simulink model "PVAndBatteryIntegratedPlantForBlackStart_SPS"  (R2024b)
settings: Solver=FixedStepAuto  StartTime=0.0  StopTime=tsim  FixedStep=Ts  RelTol=1e-9  AbsTol=1e-7
InitFcn:
  | %% Black Start Sequence
  | t0 = 0; % Battery IBR initial time
  | t1 = 0.5; % PV IBR initial time
  | t2 = 0.8; % Two IBR sync time
  | t3 = 1.2; % Additional motor load connect
  | t4 = 1.5; % Grid reconnection
  | tsim = 3.0; % Total simulation time
  | 
  | %% System Parameters
  | Vdc = 400;
  | Vnom = 100;
  | Prated = 10000;
  | Qrated = 0;
  | Srated = sqrt(Prated^2+Qrated^2);
  | wnom = 2*pi*60;
  | fnom = 60;
  | 
  | %% VOC Parameters
  | kv = Vnom;
  | ki = 3*Vnom/Srated;
  | Vminpu = 0.95;
  | dwmax = 0.5*2*pi;
  | trisemax = 0.1;
  | 
  | C = 1/sqrt(2)/Vminpu^2/dwmax;
  | L = 1/C/wnom^2;
  | tau = C/kv/ki;
  | epsilon = sqrt(L/C);
  | ksy = 3/2/trisemax;
  | 
  | V_voc_1 = 0;
  | V_voc_2 = 0;
  | 
  | %% Filter Parameters
  | Rf = 0.05;
  | Lf = 500e-6;
  | fsw = 10e3;
  | Ts = 1e-6;
  | 
  | %% Load Parameters
  | Rl = 3*Vnom^2/Prated;
  | Rl1 = Rl;
  | Rl2 = 2*Rl;
  | Rl3 = 20*Rl;
  | 
  | %% DCDC Converter Parameters
  | Kp_V = 1;
  | Ki_V = 10;
  | Imax = 110;
  | Kp_I = 0.0001;
  | Ki_I = 1;
  | Vcmax = 1;
undefined symbols (not defined in the file): C_voc, L_voc, Ll, R_voc
libraries: spsThreePhaseVIMeasurementLib x8, eeTransforms x7, spsHalfBridgeConverterLib x6, spsThreePhaseBreakerLib x6, spsThreePhaseSeriesRLCBranchLib x5, spsControlledCurrentSourceLib x4, spsControlledVoltageSourceLib x4, spsParallelRLCBranchLib x4, spsCurrentMeasurementLib x3, spsVoltageMeasurementLib x3, spsGroundLib x3, spsPower3phInstantaneousLib x3
(part 1 of 2)
settings Model: SimulationMode=accelerator  Creator=marco  LastModifiedBy=wang.shum
settings DebuggingCC: AlgebraicLoopMsg=none
settings RTWCC: GPUComputeCapability=3.5

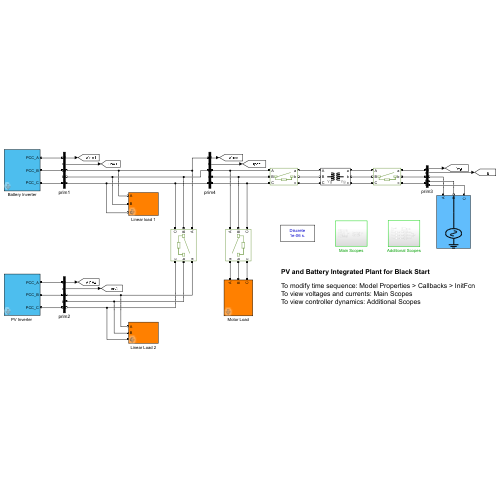
[thumbnail: Simulink's stored preview of the top-level diagram]
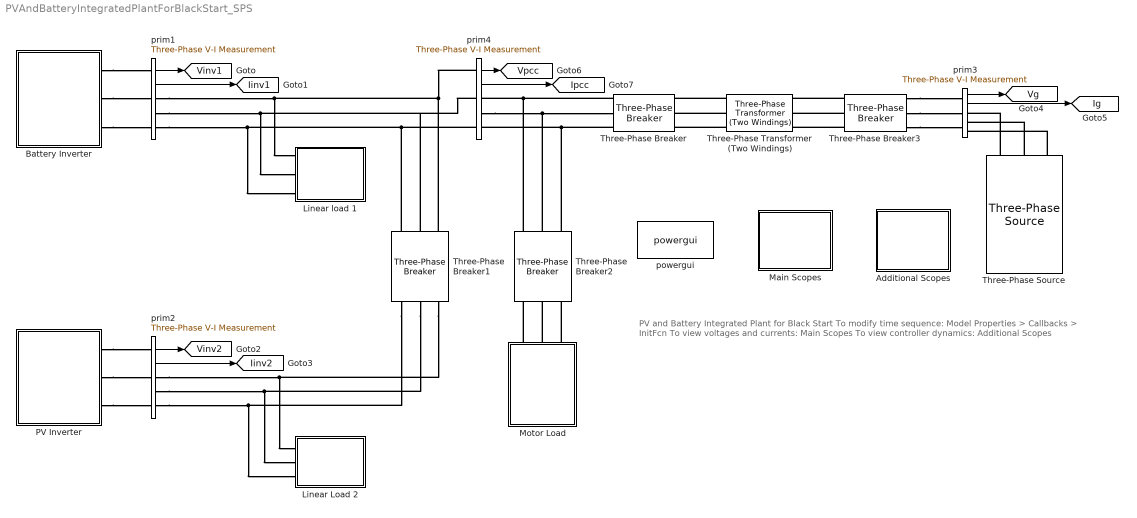
== system PVAndBatteryIntegratedPlantForBlackStart_SPS ==
  note: PV and Battery Integrated Plant for Black Start
      |
      | To modify time sequence: Model Properties > Callbacks > InitFcn
      | To view voltages and currents: Main Scopes
      | To view controller dynamics: Additional Scopes
  Additional Scopes : Subsystem
  Battery Inverter : Subsystem  mask{Vdc=Vdc, Prated=Prated, Qrated=Qrated, t0=t0}
      mask prompts: Vdc "DC Voltage"; Prated "Rated Active Power"; Qrated "Rated Reactive Power"; t0 "Enable Time"
      mask DialogControl DescTextVar Prompt: This block implements an inverter-based resource based on ideal DC source.
      mask DialogControl ParameterGroupVar Prompt: Converter Parameters
      mask DialogControl Container3 Prompt: Controller Parameters
  Linear Load 2 : Subsystem  mask{Rl2=Rl2}
      mask prompts: Rl2 "Load Resistance"
      mask DialogControl DescTextVar Prompt: This is a linear load.
  Linear load 1 : Subsystem  mask{Rl1=Rl1}
      mask prompts: Rl1 "Load Resistance"
      mask DialogControl DescTextVar Prompt: This is a linear load.
  Main Scopes : Subsystem
  Motor Load : Subsystem  mask{Rl3=Rl3, Pm=0}
      mask prompts: Rl3 "Load Resistance"; Pm "Motor Mechanical Power"
      mask DialogControl DescTextVar Prompt: This is an additional load, composed of a linear load and a motor load.
  "PV Inverter " : Subsystem  mask{Vdc=Vdc, Prated=Prated, Qrated=Qrated, t1=t1}
      mask prompts: Vdc "DC Bus Voltage"; Prated "Rated Active Power"; Qrated "Rated Reactive Power"; t1 "Enable Time"
      mask DialogControl DescTextVar Prompt: This block implements an inverter-based resource based on PV source.
      mask DialogControl ParameterGroupVar Prompt: Converter Parameters
      mask DialogControl Container3 Prompt: Controller Parameters
  Three-Phase Transformer (Two Windings) : spsThreePhaseTransformerTwoWindingsLib/Three-Phase Transformer (Two Windings)  Winding1Connection=Yg  Winding2Connection=Yg  CoreType=Three single-phase transformers  SetSaturation=off  Hysteresis=off  DataFile='hysteresis'  SetInitialFlux=off  Measurements=None  UNITS=pu  NominalPower=[ 25e3 , 60 ]  Winding1=[ 122.5 , 0.002 , 0.08 ]  Winding2=[ 122.5 , 0.002 , 0.08 ]  Rm=500  Lm=500  L0=0.5  Saturation=[ 0,0 ; 0.0024,1.2 ; 1.0,1.52 ]  InitialFluxes=[ 0.8 , -0.8 , 0.7 ]  BreakLoop=off  DiscreteSolver=Trapezoidal iterative  DataType=off  TransfoNumber=1
  Three-Phase Breaker : spsThreePhaseBreakerLib/Three-Phase Breaker  InitialState=open  SwitchA=on  SwitchB=on  SwitchC=on  SwitchTimes=t4  External=off  BreakerResistance=0.001  SnubberResistance=1e6  SnubberCapacitance=inf  Measurements=None
  Three-Phase Breaker1 : spsThreePhaseBreakerLib/Three-Phase Breaker  InitialState=open  SwitchA=on  SwitchB=on  SwitchC=on  SwitchTimes=t2  External=off  BreakerResistance=0.001  SnubberResistance=1e6  SnubberCapacitance=inf  Measurements=None
  Three-Phase Breaker2 : spsThreePhaseBreakerLib/Three-Phase Breaker  InitialState=open  SwitchA=on  SwitchB=on  SwitchC=on  SwitchTimes=t3  External=off  BreakerResistance=0.001  SnubberResistance=1e9  SnubberCapacitance=inf  Measurements=None
  Three-Phase Breaker3 : spsThreePhaseBreakerLib/Three-Phase Breaker  InitialState=open  SwitchA=on  SwitchB=on  SwitchC=on  SwitchTimes=t4  External=off  BreakerResistance=0.001  SnubberResistance=1e6  SnubberCapacitance=inf  Measurements=None
  Three-Phase Source : spsThreePhaseSourceLib/Three-Phase Source  InternalConnection=Yg  VoltagePhases=off  Voltage=Vnom*sqrt(3)  PhaseAngle=0  Voltage_phases=[25e3 25e3 25e3]/sqrt(3)  PhaseAngles_phases=[0 -120 +120]  Frequency=fnom  NonIdealSource=on  SpecifyImpedance=off  Resistance=0  Inductance=0  ShortCircuitLevel=100e6  BaseVoltage=Vnom*sqrt(3)  XRratio=7  BusType=swing  Pref=10e3  Qref=0  Prefabc=[10e3, 10e3, 10e3]  Qrefabc=[0, 0, 0]  Qmin=-inf  Qmax=inf
  powergui : sps_lib/powergui  Priority=1  SimulationMode=Discrete  SampleTime=Ts  frequency=60  Iterations=50  frequencyindice=0  Pbase=100e6  ErrMax=1e-4  UnitsV=kV  UnitsW=MW  buscounter=0  FunctionMessages=off  echomessages=off  EnableUseOfTLC=off  CurrentSourceSwitches=off  DisableSnubberDevices=off  DisableRonSwitches=off  DisableVfSwitches=off  DisplayEquations=off  AutomaticDiscreteSolvers=off  SolverType=Tustin/Backward Euler (TBE)  Interpol=off  ExternalGateDelay=off  methode=off  Ts=100  x0status=blocks  SPID=on  SwTol=0  HookPort=off  NonlinearTolerance=1e-4  nMaxIteration=100  ContinueOnMaxIteration=off  RestoreLinks=warning  ResistiveCurrentMeasurement=off  Frange=[0:2:500]  Ylog=off  Xlog=on  ShowGrid=off  save=off  variable=ZData  structure=0  ZoomFFT=off  StartTime=0.0  cycles=1  DisplayStyle=1  fundamental=60  FreqAxis=off  MaxFrequency=1000  frequencyindicesteady=1  RmsSteady=1  display=off
  prim{1..4} (4 alike) : spsThreePhaseVIMeasurementLib/Three-Phase V-I Measurement  VoltageMeasurement=phase-to-ground  SetLabelV=off  LabelV=Vabc_B1  Vpu=off  VpuLL=off  CurrentMeasurement=yes  SetLabelI=off  LabelI=Iabc_B1  Ipu=off  Pbase=100e6  Vbase=500e3  OutputType=Magnitude  PhasorSimulation=off  PSBequivalent=0
  tag scope: Ig=global, Iinv1=global, Iinv2=global, Ipcc=global, Vg=global, Vinv1=global, Vinv2=global, Vpcc=global
  wires:
  prim1/1 -> [Vinv1]
  prim1/2 -> [Iinv1]
  prim3/1 -> [Vg]
  prim3/2 -> [Ig]
  prim2/2 -> [Iinv2]
  prim2/1 -> [Vinv2]
  prim4/1 -> [Vpcc]
  prim4/2 -> [Ipcc]
  connections:
  Battery Inverter/RConn1 -- prim1/LConn1
  Battery Inverter/RConn2 -- prim1/LConn2
  Battery Inverter/RConn3 -- prim1/LConn3
  Three-Phase Breaker1/LConn3 -- prim4/LConn3 -- prim1/RConn3 -- Linear load 1/LConn3
  prim2/RConn1 -- Three-Phase Breaker1/RConn1 -- Linear Load 2/LConn1
  prim2/RConn3 -- Three-Phase Breaker1/RConn3 -- Linear Load 2/LConn3
  "PV Inverter "/RConn3 -- prim2/LConn3
  "PV Inverter "/RConn2 -- prim2/LConn2
  "PV Inverter "/RConn1 -- prim2/LConn1
  Three-Phase Source/RConn1 -- prim3/RConn1
  Three-Phase Source/RConn2 -- prim3/RConn2
  Three-Phase Source/RConn3 -- prim3/RConn3
  Three-Phase Transformer (Two Windings)/LConn2 -- Three-Phase Breaker/RConn2
  Three-Phase Transformer (Two Windings)/LConn1 -- Three-Phase Breaker/RConn1
  Three-Phase Transformer (Two Windings)/LConn3 -- Three-Phase Breaker/RConn3
  Three-Phase Breaker3/RConn2 -- prim3/LConn2
  Three-Phase Breaker3/RConn1 -- prim3/LConn1
  Three-Phase Breaker3/LConn1 -- Three-Phase Transformer (Two Windings)/RConn1
  Three-Phase Breaker3/LConn2 -- Three-Phase Transformer (Two Windings)/RConn2
  Three-Phase Breaker3/LConn3 -- Three-Phase Transformer (Two Windings)/RConn3
  Motor Load/LConn1 -- Three-Phase Breaker2/RConn1
  Motor Load/LConn2 -- Three-Phase Breaker2/RConn2
  Motor Load/LConn3 -- Three-Phase Breaker2/RConn3
  Three-Phase Breaker1/LConn1 -- prim4/LConn1 -- prim1/RConn1 -- Linear load 1/LConn1
  prim2/RConn2 -- Three-Phase Breaker1/RConn2 -- Linear Load 2/LConn2
  Three-Phase Breaker3/RConn3 -- prim3/LConn3
  prim1/RConn2 -- prim4/LConn2 -- Three-Phase Breaker1/LConn2 -- Linear load 1/LConn2
  Three-Phase Breaker2/LConn1 -- Three-Phase Breaker/LConn1 -- prim4/RConn1
  prim4/RConn2 -- Three-Phase Breaker/LConn2 -- Three-Phase Breaker2/LConn2
  Three-Phase Breaker/LConn3 -- prim4/RConn3 -- Three-Phase Breaker2/LConn3

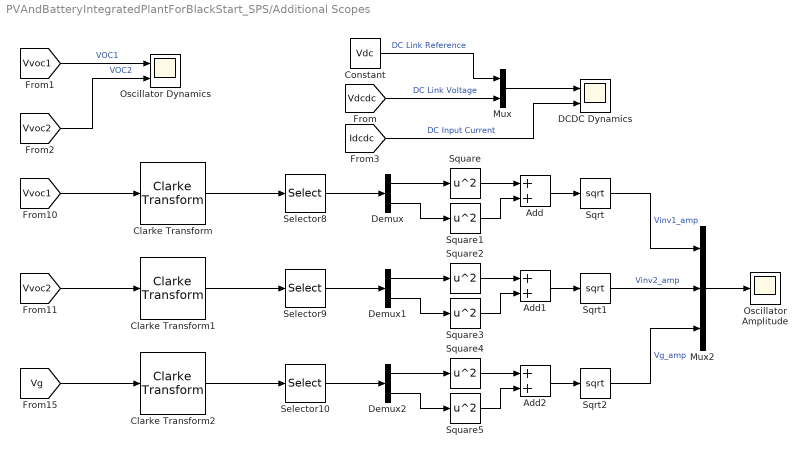
== system PVAndBatteryIntegratedPlantForBlackStart_SPS/Additional Scopes ==
  Add : Sum
  Add1 : Sum
  Add2 : Sum
  Clarke Transform : eeTransforms/Clarke Transform  PowerInvariant=off
      settings: LibrarySourceBlock=|
      | ee_sl_lib/Mathematical
      | Transforms/Clarke Transform
  Clarke Transform1 : eeTransforms/Clarke Transform  PowerInvariant=off
      settings: LibrarySourceBlock=|
      | ee_sl_lib/Mathematical
      | Transforms/Clarke Transform
  Clarke Transform2 : eeTransforms/Clarke Transform  PowerInvariant=off
      settings: LibrarySourceBlock=|
      | ee_sl_lib/Mathematical
      | Transforms/Clarke Transform
  Constant : Constant  Value=Vdc
  DCDC Dynamics : Scope  NumInputPorts=2
  Demux : Demux  Outputs=2
  Demux1 : Demux  Outputs=2
  Demux2 : Demux  Outputs=2
  Mux : Mux  Inputs=2
  Mux2 : Mux  Inputs=3
  Oscillator Amplitude : Scope
  Oscillator Dynamics : Scope  NumInputPorts=2
  Selector10 : Selector  InputPortWidth=3  IndexOptions=Index vector (dialog)  Indices=[1 2]  OutputSizes=1
  Selector8 : Selector  InputPortWidth=3  IndexOptions=Index vector (dialog)  Indices=[1 2]  OutputSizes=1
  Selector9 : Selector  InputPortWidth=3  IndexOptions=Index vector (dialog)  Indices=[1 2]  OutputSizes=1
  Sqrt : Sqrt
  Sqrt1 : Sqrt
  Sqrt2 : Sqrt
  Square{,1..5} (6 alike) : Math  Operator=square
  wires:
  Demux/1 -> Square/1
  Demux2/2 -> Square5/1
  Clarke Transform/1 -> Selector8/1
  Demux1/2 -> Square3/1
  Square1/1 -> Add/2
  [Vg] -> Clarke Transform2/1
  [Vvoc1] -> Clarke Transform/1
  Square/1 -> Add/1
  Square3/1 -> Add1/2
  Demux/2 -> Square1/1
  Selector8/1 -> Demux/1
  [Vvoc2] -> Clarke Transform1/1
  Add/1 -> Sqrt/1
  Sqrt2/1 -> Mux2/3  "Vg_amp"
  Square4/1 -> Add2/1
  Selector10/1 -> Demux2/1
  Mux2/1 -> Oscillator Amplitude/1
  Selector9/1 -> Demux1/1
  Clarke Transform1/1 -> Selector9/1
  Add1/1 -> Sqrt1/1
  Demux1/1 -> Square2/1
  Square5/1 -> Add2/2
  Sqrt1/1 -> Mux2/2  "Vinv2_amp"
  Square2/1 -> Add1/1
  Demux2/1 -> Square4/1
  Add2/1 -> Sqrt2/1
  Sqrt/1 -> Mux2/1  "Vinv1_amp"
  Clarke Transform2/1 -> Selector10/1
  [Vvoc1] -> Oscillator Dynamics/1  "VOC1"
  [Vvoc2] -> Oscillator Dynamics/2  "VOC2"
  Mux/1 -> DCDC Dynamics/1
  Constant/1 -> Mux/1  "DC Link Reference"
  [Vdcdc] -> Mux/2  "DC Link Voltage"
  [Idcdc] -> DCDC Dynamics/2  "DC Input Current"

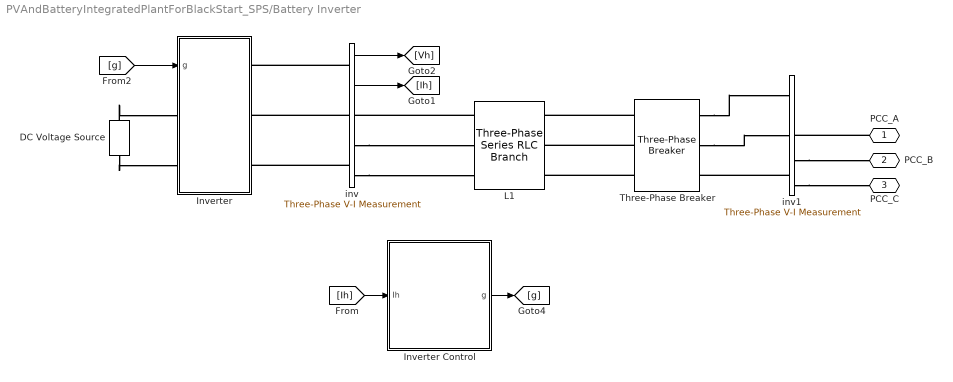
== system PVAndBatteryIntegratedPlantForBlackStart_SPS/Battery Inverter ==
  DC Voltage Source : spsDCVoltageSourceLib/DC Voltage Source  Amplitude=Vdc  Measurements=None
  Inverter : Subsystem
  Inverter Control : Subsystem
  L1 : spsThreePhaseSeriesRLCBranchLib/Three-Phase Series RLC Branch  LConnTagsString=A|B|C  RConnTagsString=A|B|C  BranchType=RL  Resistance=Rf  Inductance=Lf  Capacitance=inf  Measurements=None
  Three-Phase Breaker : spsThreePhaseBreakerLib/Three-Phase Breaker  InitialState=open  SwitchA=on  SwitchB=on  SwitchC=on  SwitchTimes=t0  External=off  BreakerResistance=0.001  SnubberResistance=1e6  SnubberCapacitance=inf  Measurements=None
  inv : spsThreePhaseVIMeasurementLib/Three-Phase V-I Measurement  VoltageMeasurement=phase-to-ground  SetLabelV=off  LabelV=Vabc_B1  Vpu=off  VpuLL=off  CurrentMeasurement=yes  SetLabelI=off  LabelI=Iabc_B1  Ipu=off  Pbase=100e6  Vbase=500e3  OutputType=Magnitude  PhasorSimulation=off  PSBequivalent=0
  inv1 : spsThreePhaseVIMeasurementLib/Three-Phase V-I Measurement  VoltageMeasurement=phase-to-ground  SetLabelV=off  LabelV=Vabc_B1  Vpu=off  VpuLL=off  CurrentMeasurement=yes  SetLabelI=off  LabelI=Iabc_B1  Ipu=off  Pbase=100e6  Vbase=500e3  OutputType=Magnitude  PhasorSimulation=off  PSBequivalent=0
  PCC_A : PMIOPort  Side=Right
  PCC_B : PMIOPort  Port=2  Side=Right
  PCC_C : PMIOPort  Port=3  Side=Right
  wires:
  [g] -> Inverter/1(g)
  inv/2 -> [Ih]
  inv/1 -> [Vh]
  [Ih] -> Inverter Control/1(Ih)
  Inverter Control/1(g) -> [g]
  connections:
  PCC_A/RConn1 -- inv1/RConn1
  inv1/RConn2 -- PCC_B/RConn1
  inv1/RConn3 -- PCC_C/RConn1
  Three-Phase Breaker/RConn1 -- inv1/LConn1
  Three-Phase Breaker/RConn2 -- inv1/LConn2
  inv1/LConn3 -- Three-Phase Breaker/RConn3
  Three-Phase Breaker/LConn3 -- L1/RConn3
  Three-Phase Breaker/LConn2 -- L1/RConn2
  Three-Phase Breaker/LConn1 -- L1/RConn1
  inv/LConn2 -- Inverter/RConn2
  L1/LConn1 -- inv/RConn1
  DC Voltage Source/RConn1 -- Inverter/LConn1
  inv/LConn3 -- Inverter/RConn3
  DC Voltage Source/LConn1 -- Inverter/LConn2
  inv/RConn3 -- L1/LConn3
  inv/LConn1 -- Inverter/RConn1
  inv/RConn2 -- L1/LConn2

== system PVAndBatteryIntegratedPlantForBlackStart_SPS/Linear Load 2 ==
  Ground1 : spsGroundLib/Ground  LConnTagsString=a
  Three-Phase Series RLC Branch1 : spsThreePhaseSeriesRLCBranchLib/Three-Phase Series RLC Branch  LConnTagsString=A|B|C  RConnTagsString=A|B|C  BranchType=R  Resistance=Rl2  Inductance=Ll  Capacitance=1e-6  Measurements=None
  A : PMIOPort  Side=Left
  B : PMIOPort  Port=2  Side=Left
  C : PMIOPort  Port=3  Side=Left
  connections:
  Three-Phase Series RLC Branch1/RConn3 -- Three-Phase Series RLC Branch1/RConn1 -- Three-Phase Series RLC Branch1/RConn2 -- Ground1/LConn1
  C/RConn1 -- Three-Phase Series RLC Branch1/LConn3
  B/RConn1 -- Three-Phase Series RLC Branch1/LConn2
  A/RConn1 -- Three-Phase Series RLC Branch1/LConn1

== system PVAndBatteryIntegratedPlantForBlackStart_SPS/Linear load 1 ==
  Ground : spsGroundLib/Ground  LConnTagsString=a
  Three-Phase Series RLC Branch : spsThreePhaseSeriesRLCBranchLib/Three-Phase Series RLC Branch  LConnTagsString=A|B|C  RConnTagsString=A|B|C  BranchType=R  Resistance=Rl1  Inductance=Ll  Capacitance=1e-6  Measurements=None
  A : PMIOPort  Side=Left
  B : PMIOPort  Port=2  Side=Left
  C : PMIOPort  Port=3  Side=Left
  connections:
  Three-Phase Series RLC Branch/RConn3 -- Ground/LConn1 -- Three-Phase Series RLC Branch/RConn2 -- Three-Phase Series RLC Branch/RConn1
  A/RConn1 -- Three-Phase Series RLC Branch/LConn1
  C/RConn1 -- Three-Phase Series RLC Branch/LConn3
  B/RConn1 -- Three-Phase Series RLC Branch/LConn2

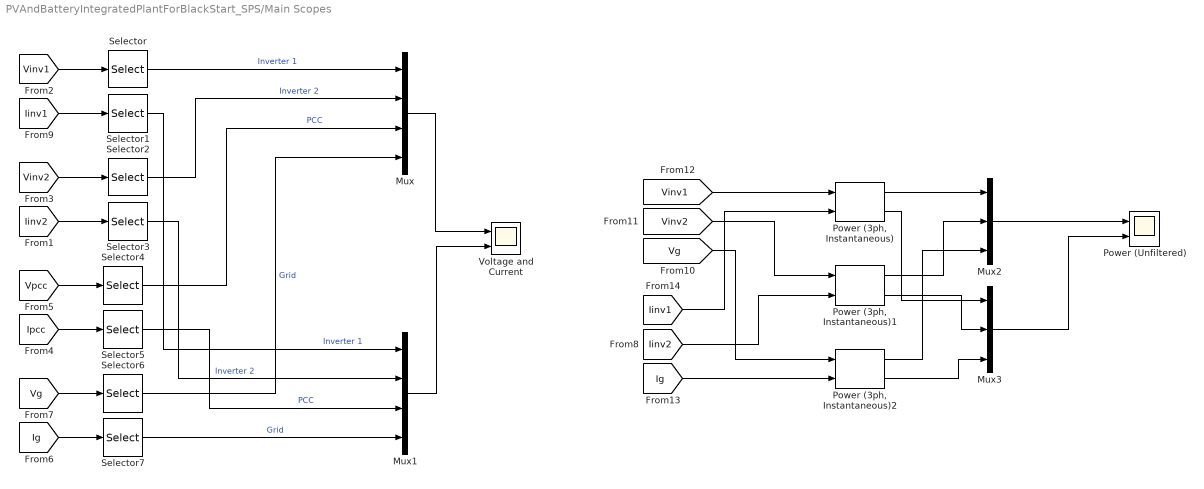
== system PVAndBatteryIntegratedPlantForBlackStart_SPS/Main Scopes ==
  Mux : Mux
  Mux1 : Mux
  Mux2 : Mux  Inputs=3
  Mux3 : Mux  Inputs=3
  "Power (3ph, Instantaneous)" : spsPower3phInstantaneousLib/Power (3ph, Instantaneous)
  "Power (3ph, Instantaneous)1" : spsPower3phInstantaneousLib/Power (3ph, Instantaneous)
  "Power (3ph, Instantaneous)2" : spsPower3phInstantaneousLib/Power (3ph, Instantaneous)
  Power (Unfiltered) : Scope  NumInputPorts=2
  Selector{,1..7} (8 alike) : Selector  InputPortWidth=3  IndexOptions=Index vector (dialog)  Indices=[1]  OutputSizes=1
  Voltage and Current : Scope  NumInputPorts=2
  wires:
  Mux/1 -> Voltage and Current/1
  Mux1/1 -> Voltage and Current/2
  [Vinv1] -> Selector/1
  [Iinv1] -> Selector1/1
  [Vinv2] -> Selector2/1
  [Iinv2] -> Selector3/1
  [Vpcc] -> Selector4/1
  [Ipcc] -> Selector5/1
  [Vg] -> Selector6/1
  [Ig] -> Selector7/1
  Selector7/1 -> Mux1/4  "Grid"
  Selector6/1 -> Mux/4  "Grid"
  Selector5/1 -> Mux1/3  "PCC"
  Selector3/1 -> Mux1/2  "Inverter 2"
  Selector1/1 -> Mux1/1  "Inverter 1"
  Selector4/1 -> Mux/3  "PCC"
  Selector2/1 -> Mux/2  "Inverter 2"
  Selector/1 -> Mux/1  "Inverter 1"
  [Iinv1] -> "Power (3ph, Instantaneous)"/2
  "Power (3ph, Instantaneous)2"/1 -> Mux2/3
  [Iinv2] -> "Power (3ph, Instantaneous)1"/2
  Mux3/1 -> Power (Unfiltered)/2
  "Power (3ph, Instantaneous)"/2 -> Mux3/1
  "Power (3ph, Instantaneous)1"/2 -> Mux3/2
  [Vg] -> "Power (3ph, Instantaneous)2"/1
  [Ig] -> "Power (3ph, Instantaneous)2"/2
  Mux2/1 -> Power (Unfiltered)/1
  [Vinv2] -> "Power (3ph, Instantaneous)1"/1
  "Power (3ph, Instantaneous)"/1 -> Mux2/1
  "Power (3ph, Instantaneous)1"/1 -> Mux2/2
  "Power (3ph, Instantaneous)2"/2 -> Mux3/3
  [Vinv1] -> "Power (3ph, Instantaneous)"/1

== system PVAndBatteryIntegratedPlantForBlackStart_SPS/Motor Load ==
  Constant : Constant  Value=Pm
  Ground2 : spsGroundLib/Ground  LConnTagsString=a
  Synchronous Machine pu Standard : spsSynchronousMachinepuStandardLib/Synchronous Machine pu Standard  PresetModel=No  MechanicalLoad=Mechanical power Pm  ShowDetailedParameters=on  RotorType=Salient-pole  Units=per unit standard parameters  MeasurementBus=off  NominalParameters=[6e+03 122.5 60]  Reactances1=[ 1.81, 0.3, 0.23, 1.76, 0.65, 0.25, 0.15 ]  Reactances2=[2.24 0.17 0.12 1.02 0.13 0.08]  dAxisTimeConstants=Short-circuit  qAxisTimeConstants=Short-circuit  TimeConstants1="[ 4.4849  0.0681  0.1  ]"  TimeConstants2=[ 8.0, 0.03, 1.0, 0.07 ]  TimeConstants3="[  4.49  0.0681  0.0513  ]"  TimeConstants4=[ 8.0, 0.03, 0.3371, 0.0295 ]  TimeConstants5=[ 1.01, 0.053, 0.1 ]  TimeConstants6=[ 1.3201, 0.023, 1.0, 0.07 ]  TimeConstants7=[0.012 0.003 0.003]  TimeConstants8=[ 1.3201, 0.0231, 0.3371, 0.0295 ]  StatorResistance=0.037875  Mechanical=[0.1028 0.02056 2]  PolePairs=20  InitialConditions="[ 0  0  0  0  0  0  0  0  1 ]"  SetSaturation=on  Saturation=[0.6404,0.7127,0.8441,0.9214,0.9956,1.082,1.19,1.316,1.457;0.7,0.7698,0.8872,0.9466,0.9969,1.046,1.1,1.151,1.201]  LoadFlowParameters=[1,0,0,0,0]  TsPowergui=0  TsBlock=-1  IterativeModel=Trapezoidal non iterative  IterativeDiscreteModel=Trapezoidal non iterative  BusType=PV  Pref=0  Qref=0  Qmin=-inf  Qmax=inf  PLF=0  QLF=0
  Terminator : Terminator
  Three-Phase Series RLC Branch3 : spsThreePhaseSeriesRLCBranchLib/Three-Phase Series RLC Branch  LConnTagsString=A|B|C  RConnTagsString=A|B|C  BranchType=R  Resistance=Rl3  Inductance=Ll  Capacitance=1e-6  Measurements=None
  A : PMIOPort  Side=Left
  B : PMIOPort  Port=2  Side=Left
  C : PMIOPort  Port=3  Side=Left
  wires:
  Synchronous Machine pu Standard/1 -> Terminator/1
  Constant/1 -> Synchronous Machine pu Standard/2, Synchronous Machine pu Standard/1
  connections:
  Three-Phase Series RLC Branch3/RConn3 -- Three-Phase Series RLC Branch3/RConn1 -- Ground2/LConn1 -- Three-Phase Series RLC Branch3/RConn2
  Three-Phase Series RLC Branch3/LConn1 -- A/RConn1 -- Synchronous Machine pu Standard/RConn1
  Synchronous Machine pu Standard/RConn2 -- B/RConn1 -- Three-Phase Series RLC Branch3/LConn2
  Three-Phase Series RLC Branch3/LConn3 -- C/RConn1 -- Synchronous Machine pu Standard/RConn3

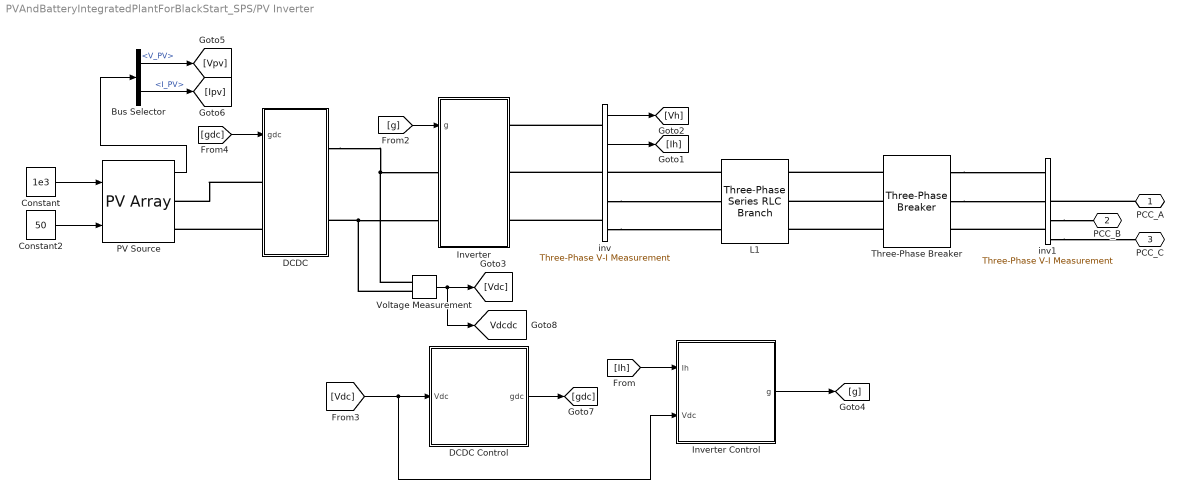
== system PVAndBatteryIntegratedPlantForBlackStart_SPS/PV Inverter  ==
  Bus Selector : BusSelector  OutputSignals=V_PV,I_PV
  Constant : Constant  Value=1e3
  Constant2 : Constant  Value=50
  DCDC : Subsystem
  DCDC Control : Subsystem  mask{Kp_V=Kp_V, Ki_V=Ki_V, Kp_I=Kp_I, Ki_I=Ki_I}
      mask prompts: Kp_V "Voltage Loop P Gain"; Ki_V "Voltage Loop I Gain"; Kp_I "Current Loop P Gain"; Ki_I "Current Loop I Gain"
      mask DialogControl DescTextVar Prompt: This is the controller for DCDC converter with PV source.
  Inverter : Subsystem
  Inverter Control : Subsystem
  L1 : spsThreePhaseSeriesRLCBranchLib/Three-Phase Series RLC Branch  LConnTagsString=A|B|C  RConnTagsString=A|B|C  BranchType=RL  Resistance=Rf  Inductance=Lf  Capacitance=inf  Measurements=None
  PV Source : spsPVArrayLib/PV Array  Npar=10  Nser=5  PlotType=array @ 1000 W/m2 & specified temperatures  S_vec="[ 1000  500  100 ]"  Temp_C_vec="[ 45 25  ]"  ModuleName=Canadian Solar Inc. CS1K-325MS  PlotWhenSelected=off  Pm=325.113  Ncell=56  Voc=37  Isc=11.31  Vm=30.7  Im=10.59  beta_Voc_pc=-0.292  alpha_Isc_pc=0.053996  beta_Voc=-0.10804  alpha_Isc=0.006107  IL=11.3215  I0=2.7652e-11  nI=0.96263  Rsh=143.3064  Rs=0.19033  RobustModel=off  RobustCellTemperature=313.3991  BAL=on  Tc=1e-6  Tfilter=5e-5
  Three-Phase Breaker : spsThreePhaseBreakerLib/Three-Phase Breaker  InitialState=open  SwitchA=on  SwitchB=on  SwitchC=on  SwitchTimes=t1  External=off  BreakerResistance=0.001  SnubberResistance=1e6  SnubberCapacitance=inf  Measurements=None
  Voltage Measurement : spsVoltageMeasurementLib/Voltage Measurement  PhasorSimulation=off  OutputType=Complex  PSBequivalent=0
  inv : spsThreePhaseVIMeasurementLib/Three-Phase V-I Measurement  VoltageMeasurement=phase-to-ground  SetLabelV=off  LabelV=Vabc_B1  Vpu=off  VpuLL=off  CurrentMeasurement=yes  SetLabelI=off  LabelI=Iabc_B1  Ipu=off  Pbase=100e6  Vbase=500e3  OutputType=Magnitude  PhasorSimulation=off  PSBequivalent=0
  inv1 : spsThreePhaseVIMeasurementLib/Three-Phase V-I Measurement  VoltageMeasurement=phase-to-ground  SetLabelV=off  LabelV=Vabc_B1  Vpu=off  VpuLL=off  CurrentMeasurement=yes  SetLabelI=off  LabelI=Iabc_B1  Ipu=off  Pbase=100e6  Vbase=500e3  OutputType=Magnitude  PhasorSimulation=off  PSBequivalent=0
  PCC_A : PMIOPort  Side=Right
  PCC_B : PMIOPort  Port=2  Side=Right
  PCC_C : PMIOPort  Port=3  Side=Right
  tag scope: Vdcdc=global
  wires:
  inv/1 -> [Vh]
  inv/2 -> [Ih]
  [g] -> Inverter/1(g)
  Voltage Measurement/1 -> [Vdcdc], [Vdc]
  Constant/1 -> PV Source/1
  Constant2/1 -> PV Source/2
  Bus Selector/1 -> [Vpv]  "<V_PV>"
  Bus Selector/2 -> [Ipv]  "<I_PV>"
  PV Source/1 -> Bus Selector/1
  DCDC Control/1(gdc) -> [gdc]
  [Ih] -> Inverter Control/1(Ih)
  [Vdc] -> Inverter Control/2(Vdc), DCDC Control/1(Vdc)
  Inverter Control/1(g) -> [g]
  [gdc] -> DCDC/1(gdc)
  connections:
  inv/RConn2 -- L1/LConn2
  inv/LConn1 -- Inverter/RConn1
  inv/RConn3 -- L1/LConn3
  inv/LConn3 -- Inverter/RConn3
  L1/LConn1 -- inv/RConn1
  inv/LConn2 -- Inverter/RConn2
  Three-Phase Breaker/LConn1 -- L1/RConn1
  Three-Phase Breaker/LConn2 -- L1/RConn2
  Three-Phase Breaker/LConn3 -- L1/RConn3
  inv1/LConn3 -- Three-Phase Breaker/RConn3
  Three-Phase Breaker/RConn2 -- inv1/LConn2
  Three-Phase Breaker/RConn1 -- inv1/LConn1
  inv1/RConn3 -- PCC_C/RConn1
  inv1/RConn2 -- PCC_B/RConn1
  PCC_A/RConn1 -- inv1/RConn1
  Voltage Measurement/LConn2 -- DCDC/RConn2 -- Inverter/LConn2
  Voltage Measurement/LConn1 -- DCDC/RConn1 -- Inverter/LConn1
  DCDC/LConn1 -- PV Source/RConn1
  DCDC/LConn2 -- PV Source/RConn2

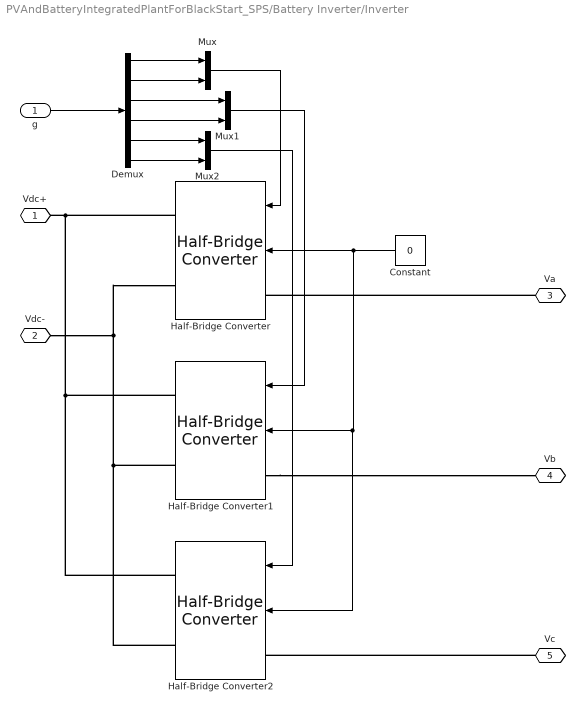
== system PVAndBatteryIntegratedPlantForBlackStart_SPS/Battery Inverter/Inverter ==
  g : Inport
  Constant : Constant  Value=0
  Demux : Demux  Outputs=6
  Half-Bridge Converter : spsHalfBridgeConverterLib/Half-Bridge Converter  ModelType=Switching devices  Ron=1e-3  Rs=1e6  Cs=inf  Vforward=[0,0]  Ron_Diode=1e-3  Rs_Diode=1e6  Cs_Diode=inf  Vf_Diode=1e-3  Rs_CurrentSource=inf  Ron_ACsource=1e-3
      settings: LibrarySourceBlock=sps_lib/Power Electronics/Half-Bridge Converter
  Half-Bridge Converter1 : spsHalfBridgeConverterLib/Half-Bridge Converter  ModelType=Switching devices  Ron=1e-3  Rs=1e6  Cs=inf  Vforward=[0,0]  Ron_Diode=1e-3  Rs_Diode=1e6  Cs_Diode=inf  Vf_Diode=1e-3  Rs_CurrentSource=inf  Ron_ACsource=1e-3
      settings: LibrarySourceBlock=sps_lib/Power Electronics/Half-Bridge Converter
  Half-Bridge Converter2 : spsHalfBridgeConverterLib/Half-Bridge Converter  ModelType=Switching devices  Ron=1e-3  Rs=1e6  Cs=inf  Vforward=[0,0]  Ron_Diode=1e-3  Rs_Diode=1e6  Cs_Diode=inf  Vf_Diode=1e-3  Rs_CurrentSource=inf  Ron_ACsource=1e-3
      settings: LibrarySourceBlock=sps_lib/Power Electronics/Half-Bridge Converter
  Mux : Mux  Inputs=2
  Mux1 : Mux  Inputs=2
  Mux2 : Mux  Inputs=2
  Vdc+ : PMIOPort  Side=Left
  Vdc- : PMIOPort  Port=2  Side=Left
  Va : PMIOPort  Port=3  Side=Right
  Vb : PMIOPort  Port=4  Side=Right
  Vc : PMIOPort  Port=5  Side=Right
  wires:
  g/1 -> Demux/1
  Constant/1 -> Half-Bridge Converter2/2, Half-Bridge Converter1/2, Half-Bridge Converter/2
  Demux/1 -> Mux/1
  Demux/2 -> Mux/2
  Demux/4 -> Mux1/2
  Demux/3 -> Mux1/1
  Demux/5 -> Mux2/1
  Demux/6 -> Mux2/2
  Mux/1 -> Half-Bridge Converter/1
  Mux1/1 -> Half-Bridge Converter1/1
  Mux2/1 -> Half-Bridge Converter2/1
  connections:
  Half-Bridge Converter/RConn1 -- Half-Bridge Converter2/RConn1 -- Half-Bridge Converter1/RConn1 -- Vdc+/RConn1
  Vdc-/RConn1 -- Half-Bridge Converter2/RConn2 -- Half-Bridge Converter1/RConn2 -- Half-Bridge Converter/RConn2
  Half-Bridge Converter1/LConn1 -- Vb/RConn1
  Vc/RConn1 -- Half-Bridge Converter2/LConn1
  Va/RConn1 -- Half-Bridge Converter/LConn1

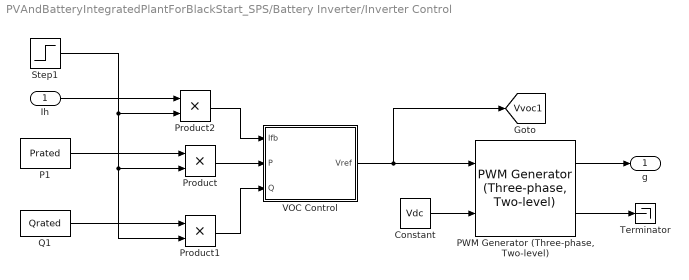
== system PVAndBatteryIntegratedPlantForBlackStart_SPS/Battery Inverter/Inverter Control ==
  Ih : Inport
  Constant : Constant  Value=Vdc
  P1 : Constant  Value=Prated
  "PWM Generator (Three-phase, Two-level)" : eePwmGeneratorTwoLevel/PWM Generator (Three-phase, Two-level)  PWMMode=Continuous PWM (CPWM)  CPWMMode=SPWM: sinusoidal PWM  DPWMMode=60 DPWM: 60 degree discontinuous PWM  fsw=fsw  Ts=Ts
      settings: LibrarySourceBlock=|
      | ee_sl_lib/Pulse Width
      | Modulation/PWM Generator
      | (Three-phase, Two-level)
  Product : Product
  Product1 : Product
  Product2 : Product
  Q1 : Constant  Value=Qrated
  Step1 : Step  Time=t0  SampleTime=0
  Terminator : Terminator
  VOC Control : Subsystem
  g : Outport
  tag scope: Vvoc1=global
  wires:
  Step1/1 -> Product2/2, Product1/2, Product/2
  "PWM Generator (Three-phase, Two-level)"/2 -> Terminator/1
  VOC Control/1(Vref) -> "PWM Generator (Three-phase, Two-level)"/1, [Vvoc1]
  Product/1 -> VOC Control/2(P)
  P1/1 -> Product/1
  Q1/1 -> Product1/1
  Product1/1 -> VOC Control/3(Q)
  Constant/1 -> "PWM Generator (Three-phase, Two-level)"/2
  Product2/1 -> VOC Control/1(Ifb)
  "PWM Generator (Three-phase, Two-level)"/1 -> g/1
  Ih/1 -> Product2/1

== system PVAndBatteryIntegratedPlantForBlackStart_SPS/PV Inverter /DCDC ==
  gdc : Inport
  Current Measurement : spsCurrentMeasurementLib/Current Measurement  PhasorSimulation=off  OutputType=Complex  PSBequivalent=0
  Diode : spsDiodeLib/Diode  Ron=0.001  Lon=0  Vf=0.8  IC=0  UseSnubber=0  Rs=500  Cs=250e-9  Measurements=off
  Mosfet : spsMosfetLib/Mosfet  Ron=0.1  Lon=0  Rd=0.01  Vfd=0  IC=0  Rs=1e5  Cs=inf  Measurements=off
  Series RLC Branch : spsSeriesRLCBranchLib/Series RLC Branch  LConnTagsString=__new0  RConnTagsString=__new0  BranchType=RL  Resistance=1e-3  Inductance=6e-4  SetiL0=off  InitialCurrent=0  Capacitance=1e-6  Setx0=off  InitialVoltage=0  Measurements=None
  Series RLC Branch1 : spsSeriesRLCBranchLib/Series RLC Branch  LConnTagsString=__new0  RConnTagsString=__new0  BranchType=RC  Resistance=1e-3  Inductance=1e-4  SetiL0=off  InitialCurrent=0  Capacitance=1e-2  Setx0=on  InitialVoltage=Vdc  Measurements=None
  Series RLC Branch2 : spsSeriesRLCBranchLib/Series RLC Branch  LConnTagsString=__new0  RConnTagsString=__new0  BranchType=RC  Resistance=1e-3  Inductance=1e-4  SetiL0=off  InitialCurrent=0  Capacitance=1e-3  Setx0=off  InitialVoltage=Vdc  Measurements=None
  DC+ : PMIOPort  Side=Right
  PV+ : PMIOPort  Port=2  Side=Left
  PV- : PMIOPort  Port=3  Side=Left
  DC- : PMIOPort  Port=4  Side=Right
  tag scope: Idcdc=global
  wires:
  gdc/1 -> Mosfet/1
  Current Measurement/1 -> [Idcdc]
  connections:
  Mosfet/LConn1 -- Diode/LConn1 -- Current Measurement/RConn1
  Series RLC Branch/LConn1 -- Series RLC Branch2/LConn1 -- PV+/RConn1
  Series RLC Branch1/LConn1 -- DC+/RConn1 -- Diode/RConn1
  Series RLC Branch2/RConn1 -- DC-/RConn1 -- Series RLC Branch1/RConn1 -- Mosfet/RConn1 -- PV-/RConn1
  Current Measurement/LConn1 -- Series RLC Branch/RConn1

== system PVAndBatteryIntegratedPlantForBlackStart_SPS/PV Inverter /DCDC Control ==
  Vdc : Inport
  Constant3 : Constant  Value=Vdc
  PID Controller : slpidlib/PID Controller  Controller=PI  Form=Parallel  TimeDomain=Discrete-time  UseExternalTs=off  SampleTime=-1  IntegratorMethod=Forward Euler  FilterMethod=Forward Euler  ControllerParametersSource=internal  P=Kp_V  I=Ki_V  UseKiTs=off  D=0  UseExternalDerivativeSource=off  N=100  UseFilter=on  TunerSelectOption=Transfer Function Based (PID Tuner App)  InitialConditionSource=internal  InitialConditionForIntegrator=0  InitialConditionForFilter=0  DifferentiatorICPrevScaledInput=0  ExternalReset=none  TrackingMode=off  Kt=1  LimitOutput=on  SatLimitsSource=internal  UpperSaturationLimit=Imax  LowerSaturationLimit=0  LinearizeAsGain=on  AntiWindupMode=back-calculation  Kb=1  LimitIntegrator=off  UpperIntegratorSaturationLimit=inf  LowerIntegratorSaturationLimit=-inf  POutMin=[]  POutMax=[]  IOutMin=[]  IOutMax=[]  DOutMin=[]  DOutMax=[]  NOutMin=[]  NOutMax=[]  SumOutMin=[]  SumOutMax=[]  SaturationOutMin=[]  SaturationOutMax=[]  PParamMin=[]  PParamMax=[]  IParamMin=[]  IParamMax=[]  DParamMin=[]  DParamMax=[]  NParamMin=[]  NParamMax=[]  KbParamMin=[]  KbParamMax=[]  KtParamMin=[]  KtParamMax=[]  KbOutMin=[]  KbOutMax=[]  KtOutMin=[]  KtOutMax=[]  IntegratorOutMin=[]  IntegratorOutMax=[]  FilterOutMin=[]  FilterOutMax=[]  SumI1OutMin=[]  SumI1OutMax=[]  SumI2OutMin=[]  SumI2OutMax=[]  SumI3OutMin=[]  SumI3OutMax=[]  SumI4OutMin=[]  SumI4OutMax=[]  SumDOutMin=[]  SumDOutMax=[]  DifferentiatorOutMin=[]  DifferentiatorOutMax=[]  FilterDiffOutCoefMin=[]  FilterDiffOutCoefMax=[]  ReciprocalOutMin=[]  ReciprocalOutMax=[]  SumDenOutMin=[]  SumDenOutMax=[]  SumNumOutMin=[]  SumNumOutMax=[]  DivideOutMin=[]  DivideOutMax=[]  UdiffTsProdOutMin=[]  UdiffTsProdOutMax=[]  NTsProdOutMin=[]  NTsProdOutMax=[]  UintegralTsProdOutMin=[]  UintegralTsProdOutMax=[]  UngainTsProdOutMin=[]  UngainTsProdOutMax=[]  ClampingZeroOutDataTypeStr=Inherit: Inherit via back propagation  ClampingZeroOutMin=[]  ClampingZeroOutMax=[]  FilterDenConstantOutDataTypeStr=Inherit: Inherit via back propagation  FilterDenConstantOutMin=[]  FilterDenConstantOutMax=[]  PCopyOutDataTypeStr=Inherit: Inherit via back propagation  PCopyOutMin=[]  PCopyOutMax=[]  NCopyOutDataTypeStr=Inherit: Inherit via back propagation  NCopyOutMin=[]  NCopyOutMax=[]  IntegratorContinuousStateAttributes=''  IntegratorStateMustResolveToSignalObject=off  IntegratorRTWStateStorageClass=Auto  FilterContinuousStateAttributes=''  FilterStateMustResolveToSignalObject=off  FilterRTWStateStorageClass=Auto  ParallelPVariant=InternalParameters  IdealPVariant=Disabled  IVariant=InternalParameters  DVariant=Disabled  IntegratorVariant=Discrete  SatVariant=Enabled  AWVariant=BackCalculation  PCopyVariant=Disabled  TRVariant=Disabled  FdbkBlocksVariant=Forward  IdealPFdbkVariant=Disabled  SatFdbkVariant=Disabled  DerivativeFilterVariant=Disabled  NVariant=Disabled  NCopyVariant=Disabled_SignalSpec  FilterICVariant=Disabled  IntegratorICVariant=InternalICs  ExternalResetVariant=Disabled  TRSumVariant=Passthrough  SumFdbkVariant=Disabled  SumVariant=Sum_PI  TsampFilterVariant=InternalTs  TsampNgainVariant=Passthrough  TsampIntegralVariant=Disabled_SignalSpec  ExternalSaturationOutDataTypeStr=Inherit: Same as second input  DerivativeSourceVariant=Disabled  PreIntVariant=InternalPreInt
  PID Controller1 : slpidlib/PID Controller  Controller=PI  Form=Parallel  TimeDomain=Discrete-time  UseExternalTs=off  SampleTime=-1  IntegratorMethod=Forward Euler  FilterMethod=Forward Euler  ControllerParametersSource=internal  P=Kp_I  I=Ki_I  UseKiTs=off  D=0  UseExternalDerivativeSource=off  N=100  UseFilter=on  TunerSelectOption=Transfer Function Based (PID Tuner App)  InitialConditionSource=internal  InitialConditionForIntegrator=0  InitialConditionForFilter=0  DifferentiatorICPrevScaledInput=0  ExternalReset=none  TrackingMode=off  Kt=1  LimitOutput=on  SatLimitsSource=internal  UpperSaturationLimit=Vcmax  LowerSaturationLimit=0  LinearizeAsGain=on  AntiWindupMode=back-calculation  Kb=1  LimitIntegrator=off  UpperIntegratorSaturationLimit=inf  LowerIntegratorSaturationLimit=-inf  POutMin=[]  POutMax=[]  IOutMin=[]  IOutMax=[]  DOutMin=[]  DOutMax=[]  NOutMin=[]  NOutMax=[]  SumOutMin=[]  SumOutMax=[]  SaturationOutMin=[]  SaturationOutMax=[]  PParamMin=[]  PParamMax=[]  IParamMin=[]  IParamMax=[]  DParamMin=[]  DParamMax=[]  NParamMin=[]  NParamMax=[]  KbParamMin=[]  KbParamMax=[]  KtParamMin=[]  KtParamMax=[]  KbOutMin=[]  KbOutMax=[]  KtOutMin=[]  KtOutMax=[]  IntegratorOutMin=[]  IntegratorOutMax=[]  FilterOutMin=[]  FilterOutMax=[]  SumI1OutMin=[]  SumI1OutMax=[]  SumI2OutMin=[]  SumI2OutMax=[]  SumI3OutMin=[]  SumI3OutMax=[]  SumI4OutMin=[]  SumI4OutMax=[]  SumDOutMin=[]  SumDOutMax=[]  DifferentiatorOutMin=[]  DifferentiatorOutMax=[]  FilterDiffOutCoefMin=[]  FilterDiffOutCoefMax=[]  ReciprocalOutMin=[]  ReciprocalOutMax=[]  SumDenOutMin=[]  SumDenOutMax=[]  SumNumOutMin=[]  SumNumOutMax=[]  DivideOutMin=[]  DivideOutMax=[]  UdiffTsProdOutMin=[]  UdiffTsProdOutMax=[]  NTsProdOutMin=[]  NTsProdOutMax=[]  UintegralTsProdOutMin=[]  UintegralTsProdOutMax=[]  UngainTsProdOutMin=[]  UngainTsProdOutMax=[]  ClampingZeroOutDataTypeStr=Inherit: Inherit via back propagation  ClampingZeroOutMin=[]  ClampingZeroOutMax=[]  FilterDenConstantOutDataTypeStr=Inherit: Inherit via back propagation  FilterDenConstantOutMin=[]  FilterDenConstantOutMax=[]  PCopyOutDataTypeStr=Inherit: Inherit via back propagation  PCopyOutMin=[]  PCopyOutMax=[]  NCopyOutDataTypeStr=Inherit: Inherit via back propagation  NCopyOutMin=[]  NCopyOutMax=[]  IntegratorContinuousStateAttributes=''  IntegratorStateMustResolveToSignalObject=off  IntegratorRTWStateStorageClass=Auto  FilterContinuousStateAttributes=''  FilterStateMustResolveToSignalObject=off  FilterRTWStateStorageClass=Auto  ParallelPVariant=InternalParameters  IdealPVariant=Disabled  IVariant=InternalParameters  DVariant=Disabled  IntegratorVariant=Discrete  SatVariant=Enabled  AWVariant=BackCalculation  PCopyVariant=Disabled  TRVariant=Disabled  FdbkBlocksVariant=Forward  IdealPFdbkVariant=Disabled  SatFdbkVariant=Disabled  DerivativeFilterVariant=Disabled  NVariant=Disabled  NCopyVariant=Disabled_SignalSpec  FilterICVariant=Disabled  IntegratorICVariant=InternalICs  ExternalResetVariant=Disabled  TRSumVariant=Passthrough  SumFdbkVariant=Disabled  SumVariant=Sum_PI  TsampFilterVariant=InternalTs  TsampNgainVariant=Passthrough  TsampIntegralVariant=Disabled_SignalSpec  ExternalSaturationOutDataTypeStr=Inherit: Same as second input  DerivativeSourceVariant=Disabled  PreIntVariant=InternalPreInt
  PWM Generator (DC-DC) : spsPWMGeneratorDCDCLib/PWM Generator (DC-DC)  Fsw=fsw  Ts=Ts
  Subtract : Sum  Inputs=+-
  Subtract2 : Sum  Inputs=+-
  gdc : Outport
  wires:
  PID Controller1/1 -> PWM Generator (DC-DC)/1
  Subtract/1 -> PID Controller/1
  Subtract2/1 -> PID Controller1/1
  [Idcdc] -> Subtract2/2
  Vdc/1 -> Subtract/2
  PID Controller/1 -> Subtract2/1
  PWM Generator (DC-DC)/1 -> gdc/1
  Constant3/1 -> Subtract/1

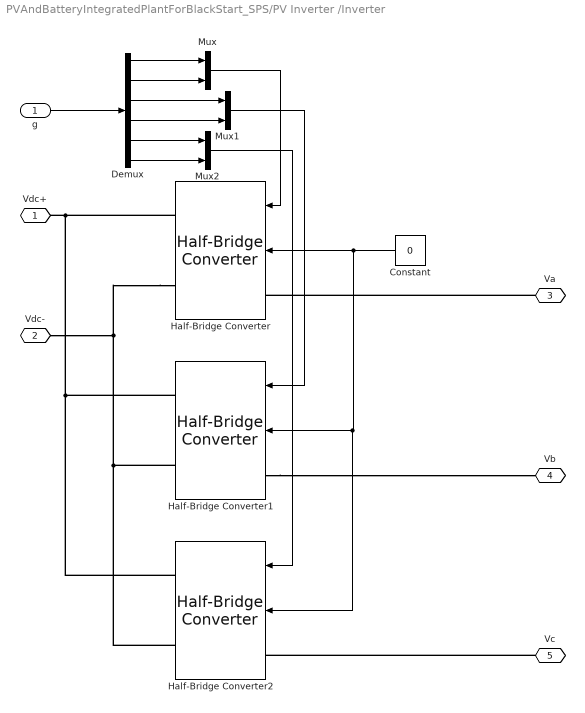
== system PVAndBatteryIntegratedPlantForBlackStart_SPS/PV Inverter /Inverter ==
  g : Inport
  Constant : Constant  Value=0
  Demux : Demux  Outputs=6
  Half-Bridge Converter : spsHalfBridgeConverterLib/Half-Bridge Converter  ModelType=Switching devices  Ron=1e-3  Rs=1e6  Cs=inf  Vforward=[0,0]  Ron_Diode=1e-3  Rs_Diode=1e6  Cs_Diode=inf  Vf_Diode=1e-3  Rs_CurrentSource=inf  Ron_ACsource=1e-3
  Half-Bridge Converter1 : spsHalfBridgeConverterLib/Half-Bridge Converter  ModelType=Switching devices  Ron=1e-3  Rs=1e6  Cs=inf  Vforward=[0,0]  Ron_Diode=1e-3  Rs_Diode=1e6  Cs_Diode=inf  Vf_Diode=1e-3  Rs_CurrentSource=inf  Ron_ACsource=1e-3
  Half-Bridge Converter2 : spsHalfBridgeConverterLib/Half-Bridge Converter  ModelType=Switching devices  Ron=1e-3  Rs=1e6  Cs=inf  Vforward=[0,0]  Ron_Diode=1e-3  Rs_Diode=1e6  Cs_Diode=inf  Vf_Diode=1e-3  Rs_CurrentSource=inf  Ron_ACsource=1e-3
  Mux : Mux  Inputs=2
  Mux1 : Mux  Inputs=2
  Mux2 : Mux  Inputs=2
  Vdc+ : PMIOPort  Side=Left
  Vdc- : PMIOPort  Port=2  Side=Left
  Va : PMIOPort  Port=3  Side=Right
  Vb : PMIOPort  Port=4  Side=Right
  Vc : PMIOPort  Port=5  Side=Right
  wires:
  Mux2/1 -> Half-Bridge Converter2/1
  Mux1/1 -> Half-Bridge Converter1/1
  Mux/1 -> Half-Bridge Converter/1
  Demux/6 -> Mux2/2
  Demux/5 -> Mux2/1
  Demux/3 -> Mux1/1
  Demux/4 -> Mux1/2
  Demux/2 -> Mux/2
  Demux/1 -> Mux/1
  Constant/1 -> Half-Bridge Converter/2, Half-Bridge Converter1/2, Half-Bridge Converter2/2
  g/1 -> Demux/1
  connections:
  Va/RConn1 -- Half-Bridge Converter/LConn1
  Vc/RConn1 -- Half-Bridge Converter2/LConn1
  Half-Bridge Converter1/LConn1 -- Vb/RConn1
  Half-Bridge Converter/RConn2 -- Half-Bridge Converter1/RConn2 -- Half-Bridge Converter2/RConn2 -- Vdc-/RConn1
  Vdc+/RConn1 -- Half-Bridge Converter1/RConn1 -- Half-Bridge Converter2/RConn1 -- Half-Bridge Converter/RConn1

== system PVAndBatteryIntegratedPlantForBlackStart_SPS/PV Inverter /Inverter Control ==
  Ih : Inport
  Vdc : Inport  Port=2
  P2 : Constant  Value=Prated
  "PWM Generator (Three-phase, Two-level)" : eePwmGeneratorTwoLevel/PWM Generator (Three-phase, Two-level)  PWMMode=Continuous PWM (CPWM)  CPWMMode=SPWM: sinusoidal PWM  DPWMMode=60 DPWM: 60 degree discontinuous PWM  fsw=fsw  Ts=Ts
  Product : Product
  Product1 : Product
  Product2 : Product
  Q2 : Constant  Value=Qrated
  Step2 : Step  Time=t1  SampleTime=0
  Terminator : Terminator
  VOC Control : Subsystem
  g : Outport
  tag scope: Vvoc2=global
  wires:
  Step2/1 -> Product2/2, Product/2, Product1/2
  Vdc/1 -> "PWM Generator (Three-phase, Two-level)"/2
  P2/1 -> Product/1
  Q2/1 -> Product1/1
  Product/1 -> VOC Control/2(P)
  Product1/1 -> VOC Control/3(Q)
  Ih/1 -> Product2/1
  VOC Control/1(Vref) -> "PWM Generator (Three-phase, Two-level)"/1, [Vvoc2]
  "PWM Generator (Three-phase, Two-level)"/2 -> Terminator/1
  Product2/1 -> VOC Control/1(Ifb)
  "PWM Generator (Three-phase, Two-level)"/1 -> g/1

== system PVAndBatteryIntegratedPlantForBlackStart_SPS/Battery Inverter/Inverter Control/VOC Control ==
  Ifb : Inport
  P : Inport  Port=2
  Q : Inport  Port=3
  Constant : Constant  Value=0
  Inverse Clarke Transform : eeTransforms/Inverse Clarke Transform  PowerInvariant=off
      settings: LibrarySourceBlock=|
      | ee_sl_lib/Mathematical
      | Transforms/Inverse
      | Clarke Transform
  Memory : Memory
  Memory1 : Memory
  Mux1 : Mux  Inputs=3
  Subsystem : Subsystem
  VOC_DE : Subsystem
  Vref : Outport
  wires:
  Memory1/1 -> Subsystem/5(vbe)
  Memory/1 -> Subsystem/4(val)
  Mux1/1 -> Inverse Clarke Transform/1
  Ifb/1 -> Subsystem/1(If)
  Inverse Clarke Transform/1 -> Vref/1
  VOC_DE/1(val) -> Memory/1, Mux1/1
  VOC_DE/2(vbe) -> Mux1/2, Memory1/1
  Constant/1 -> Mux1/3
  Subsystem/1(u) -> VOC_DE/1(u)
  P/1 -> Subsystem/2(P)
  Q/1 -> Subsystem/3(Q)

== system PVAndBatteryIntegratedPlantForBlackStart_SPS/PV Inverter /Inverter Control/VOC Control ==
  Ifb : Inport
  P : Inport  Port=2
  Q : Inport  Port=3
  Constant : Constant  Value=0
  Inverse Clarke Transform : eeTransforms/Inverse Clarke Transform  PowerInvariant=off
      settings: LibrarySourceBlock=|
      | ee_sl_lib/Mathematical
      | Transforms/Inverse
      | Clarke Transform
  Memory : Memory
  Memory1 : Memory
  Mux1 : Mux  Inputs=3
  Subsystem : Subsystem
  VOC_DE : Subsystem
  Vref : Outport
  wires:
  Q/1 -> Subsystem/3(Q)
  P/1 -> Subsystem/2(P)
  Subsystem/1(u) -> VOC_DE/1(u)
  Constant/1 -> Mux1/3
  VOC_DE/2(vbe) -> Memory1/1, Mux1/2
  VOC_DE/1(val) -> Mux1/1, Memory/1
  Inverse Clarke Transform/1 -> Vref/1
  Ifb/1 -> Subsystem/1(If)
  Mux1/1 -> Inverse Clarke Transform/1
  Memory/1 -> Subsystem/4(val)
  Memory1/1 -> Subsystem/5(vbe)

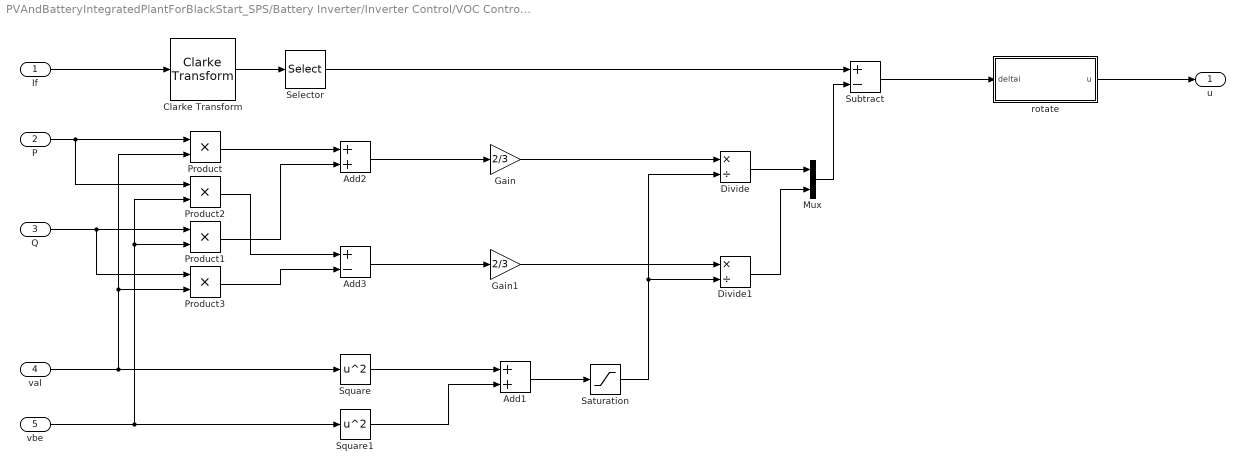
== system PVAndBatteryIntegratedPlantForBlackStart_SPS/Battery Inverter/Inverter Control/VOC Control/Subsystem ==
  If : Inport
  P : Inport  Port=2
  Q : Inport  Port=3
  val : Inport  Port=4
  vbe : Inport  Port=5
  Add1 : Sum
  Add2 : Sum
  Add3 : Sum  Inputs=+-
  Clarke Transform : eeTransforms/Clarke Transform  PowerInvariant=off
      settings: LibrarySourceBlock=|
      | ee_sl_lib/Mathematical
      | Transforms/Clarke Transform
  Divide : Product  Inputs=*/
  Divide1 : Product  Inputs=*/
  Gain : Gain  Gain=2/3
  Gain1 : Gain  Gain=2/3
  Mux : Mux  Inputs=2
  Product{,1..3} (4 alike) : Product
  Saturation : Saturate  UpperLimit=inf  LowerLimit=1e-9
  Selector : Selector  InputPortWidth=3  IndexOptions=Index vector (dialog)  Indices=[1 2]  OutputSizes=1
  Square : Math  Operator=square
  Square1 : Math  Operator=square
  Subtract : Sum  Inputs=+-
  rotate : Subsystem
  u : Outport
  wires:
  Clarke Transform/1 -> Selector/1
  If/1 -> Clarke Transform/1
  val/1 -> Product3/2, Product/2, Square/1
  vbe/1 -> Product2/2, Product1/2, Square1/1
  Square/1 -> Add1/1
  Square1/1 -> Add1/2
  Selector/1 -> Subtract/1
  Add1/1 -> Saturation/1
  P/1 -> Product2/1, Product/1
  Q/1 -> Product3/1, Product1/1
  Product/1 -> Add2/1
  Product1/1 -> Add2/2
  Add2/1 -> Gain/1
  Gain/1 -> Divide/1
  Saturation/1 -> Divide/2, Divide1/2
  Product2/1 -> Add3/1
  Product3/1 -> Add3/2
  Add3/1 -> Gain1/1
  Gain1/1 -> Divide1/1
  Divide/1 -> Mux/1
  Divide1/1 -> Mux/2
  Mux/1 -> Subtract/2
  Subtract/1 -> rotate/1(deltai)
  rotate/1(u) -> u/1

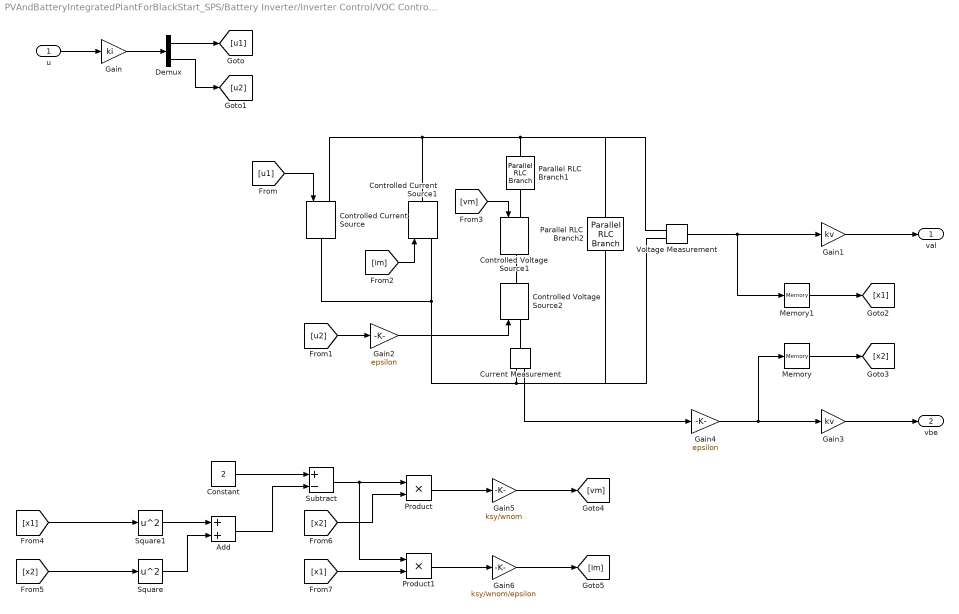
== system PVAndBatteryIntegratedPlantForBlackStart_SPS/Battery Inverter/Inverter Control/VOC Control/VOC_DE ==
  u : Inport
  Add : Sum
  Constant : Constant  Value=2
  Controlled Current Source : spsControlledCurrentSourceLib/Controlled Current Source  Initialize=off  Source_Type=AC  Amplitude=0  Phase=0  Frequency=0  Measurements=None
  Controlled Current Source1 : spsControlledCurrentSourceLib/Controlled Current Source  Initialize=off  Source_Type=AC  Amplitude=0  Phase=0  Frequency=0  Measurements=None
  Controlled Voltage Source1 : spsControlledVoltageSourceLib/Controlled Voltage Source  Initialize=on  Source_Type=DC  Amplitude=0  Phase=0  Frequency=0  Measurements=None
  Controlled Voltage Source2 : spsControlledVoltageSourceLib/Controlled Voltage Source  Initialize=on  Source_Type=DC  Amplitude=0  Phase=0  Frequency=0  Measurements=None
  Current Measurement : spsCurrentMeasurementLib/Current Measurement  PhasorSimulation=off  OutputType=Complex  PSBequivalent=0
  Demux : Demux  Outputs=2
  Gain : Gain  Gain=ki
  Gain1 : Gain  Gain=kv
  Gain2 : Gain  Gain=epsilon
  Gain3 : Gain  Gain=kv
  Gain4 : Gain  Gain=epsilon
  Gain5 : Gain  Gain=ksy/wnom
  Gain6 : Gain  Gain=ksy/wnom/epsilon
  Memory : Memory
  Memory1 : Memory
  Parallel RLC Branch1 : spsParallelRLCBranchLib/Parallel RLC Branch  LConnTagsString=a  RConnTagsString=__new0  BranchType=L  Resistance=R_voc  Inductance=L  SetiL0=on  InitialCurrent=0  Capacitance=C_voc  Setx0=off  InitialVoltage=0  Measurements=None
  Parallel RLC Branch2 : spsParallelRLCBranchLib/Parallel RLC Branch  LConnTagsString=a  RConnTagsString=__new0  BranchType=C  Resistance=R_voc  Inductance=L_voc  SetiL0=off  InitialCurrent=0  Capacitance=C  Setx0=on  InitialVoltage=V_voc_1  Measurements=None
  Product : Product
  Product1 : Product
  Square : Math  Operator=square
  Square1 : Math  Operator=square
  Subtract : Sum  Inputs=+-
  Voltage Measurement : spsVoltageMeasurementLib/Voltage Measurement  PhasorSimulation=off  OutputType=Complex  PSBequivalent=0
  val : Outport
  vbe : Outport  Port=2
  wires:
  Memory1/1 -> [x1]
  Memory/1 -> [x2]
  [x2] -> Square/1
  [x1] -> Square1/1
  u/1 -> Gain/1
  Voltage Measurement/1 -> Gain1/1, Memory1/1
  Gain1/1 -> val/1
  Gain/1 -> Demux/1
  Demux/1 -> [u1]
  Demux/2 -> [u2]
  [u1] -> Controlled Current Source/1
  [u2] -> Gain2/1
  Gain2/1 -> Controlled Voltage Source2/1
  [im] -> Controlled Current Source1/1
  [vm] -> Controlled Voltage Source1/1
  Gain3/1 -> vbe/1
  Gain4/1 -> Gain3/1, Memory/1
  Current Measurement/1 -> Gain4/1
  Constant/1 -> Subtract/1
  Square1/1 -> Add/1
  Square/1 -> Add/2
  Add/1 -> Subtract/2
  Subtract/1 -> Product1/1, Product/1
  [x2] -> Product/2
  Product/1 -> Gain5/1
  Gain5/1 -> [vm]
  [x1] -> Product1/2
  Product1/1 -> Gain6/1
  Gain6/1 -> [im]
  connections:
  Controlled Current Source1/LConn1 -- Controlled Current Source/RConn1 -- Current Measurement/RConn1 -- Parallel RLC Branch2/RConn1 -- Voltage Measurement/LConn2
  Controlled Current Source/LConn1 -- Controlled Current Source1/RConn1 -- Parallel RLC Branch1/LConn1 -- Parallel RLC Branch2/LConn1 -- Voltage Measurement/LConn1
  Controlled Voltage Source1/LConn1 -- Parallel RLC Branch1/RConn1
  Controlled Voltage Source2/RConn1 -- Controlled Voltage Source1/RConn1
  Controlled Voltage Source2/LConn1 -- Current Measurement/LConn1

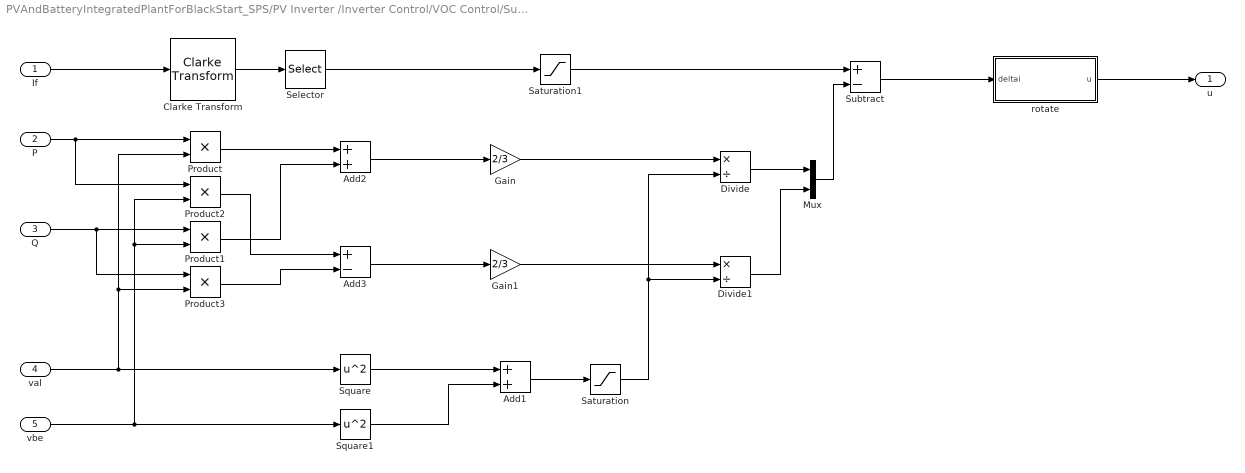
== system PVAndBatteryIntegratedPlantForBlackStart_SPS/PV Inverter /Inverter Control/VOC Control/Subsystem ==
  If : Inport
  P : Inport  Port=2
  Q : Inport  Port=3
  val : Inport  Port=4
  vbe : Inport  Port=5
  Add1 : Sum
  Add2 : Sum
  Add3 : Sum  Inputs=+-
  Clarke Transform : eeTransforms/Clarke Transform  PowerInvariant=off
      settings: LibrarySourceBlock=|
      | ee_sl_lib/Mathematical
      | Transforms/Clarke Transform
  Divide : Product  Inputs=*/
  Divide1 : Product  Inputs=*/
  Gain : Gain  Gain=2/3
  Gain1 : Gain  Gain=2/3
  Mux : Mux  Inputs=2
  Product{,1..3} (4 alike) : Product
  Saturation : Saturate  UpperLimit=inf  LowerLimit=1e-9
  Saturation1 : Saturate  UpperLimit=1e3  LowerLimit=-1e3
  Selector : Selector  InputPortWidth=3  IndexOptions=Index vector (dialog)  Indices=[1 2]  OutputSizes=1
  Square : Math  Operator=square
  Square1 : Math  Operator=square
  Subtract : Sum  Inputs=+-
  rotate : Subsystem
  u : Outport
  wires:
  rotate/1(u) -> u/1
  Subtract/1 -> rotate/1(deltai)
  Mux/1 -> Subtract/2
  Divide1/1 -> Mux/2
  Divide/1 -> Mux/1
  Gain1/1 -> Divide1/1
  Add3/1 -> Gain1/1
  Product3/1 -> Add3/2
  Product2/1 -> Add3/1
  Saturation/1 -> Divide1/2, Divide/2
  Gain/1 -> Divide/1
  Add2/1 -> Gain/1
  Product1/1 -> Add2/2
  Product/1 -> Add2/1
  Q/1 -> Product1/1, Product3/1
  P/1 -> Product/1, Product2/1
  Add1/1 -> Saturation/1
  Square1/1 -> Add1/2
  Square/1 -> Add1/1
  vbe/1 -> Square1/1, Product1/2, Product2/2
  val/1 -> Square/1, Product/2, Product3/2
  If/1 -> Clarke Transform/1
  Clarke Transform/1 -> Selector/1
  Selector/1 -> Saturation1/1
  Saturation1/1 -> Subtract/1

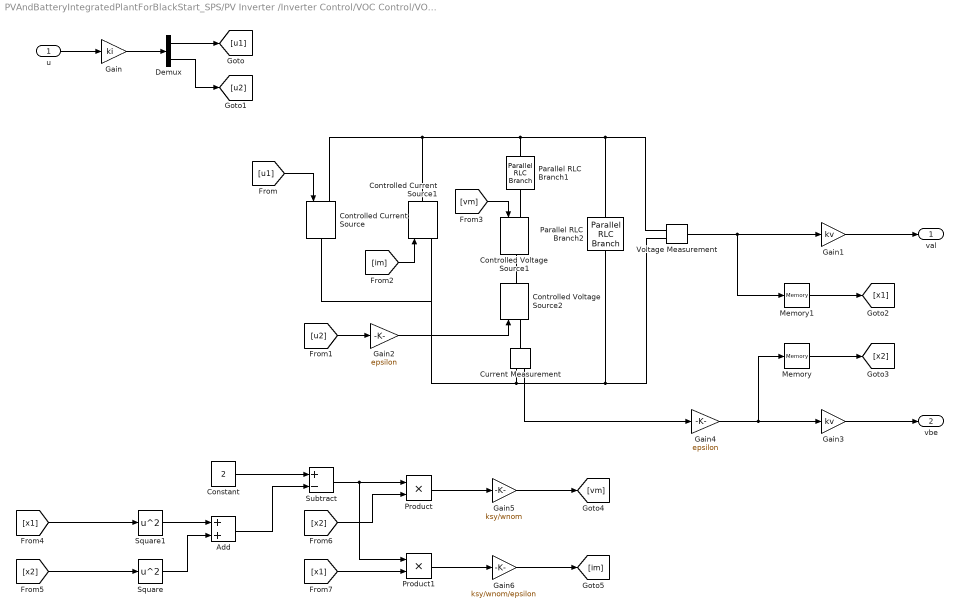
== system PVAndBatteryIntegratedPlantForBlackStart_SPS/PV Inverter /Inverter Control/VOC Control/VOC_DE ==
  u : Inport
  Add : Sum
  Constant : Constant  Value=2
  Controlled Current Source : spsControlledCurrentSourceLib/Controlled Current Source  Initialize=off  Source_Type=AC  Amplitude=0  Phase=0  Frequency=0  Measurements=None
  Controlled Current Source1 : spsControlledCurrentSourceLib/Controlled Current Source  Initialize=off  Source_Type=AC  Amplitude=0  Phase=0  Frequency=0  Measurements=None
  Controlled Voltage Source1 : spsControlledVoltageSourceLib/Controlled Voltage Source  Initialize=on  Source_Type=DC  Amplitude=0  Phase=0  Frequency=0  Measurements=None
  Controlled Voltage Source2 : spsControlledVoltageSourceLib/Controlled Voltage Source  Initialize=on  Source_Type=DC  Amplitude=0  Phase=0  Frequency=0  Measurements=None
  Current Measurement : spsCurrentMeasurementLib/Current Measurement  PhasorSimulation=off  OutputType=Complex  PSBequivalent=0
  Demux : Demux  Outputs=2
  Gain : Gain  Gain=ki
  Gain1 : Gain  Gain=kv
  Gain2 : Gain  Gain=epsilon
  Gain3 : Gain  Gain=kv
  Gain4 : Gain  Gain=epsilon
  Gain5 : Gain  Gain=ksy/wnom
  Gain6 : Gain  Gain=ksy/wnom/epsilon
  Memory : Memory
  Memory1 : Memory
  Parallel RLC Branch1 : spsParallelRLCBranchLib/Parallel RLC Branch  LConnTagsString=a  RConnTagsString=__new0  BranchType=L  Resistance=R_voc  Inductance=L  SetiL0=on  InitialCurrent=0  Capacitance=C_voc  Setx0=off  InitialVoltage=0  Measurements=None
  Parallel RLC Branch2 : spsParallelRLCBranchLib/Parallel RLC Branch  LConnTagsString=a  RConnTagsString=__new0  BranchType=C  Resistance=R_voc  Inductance=L_voc  SetiL0=off  InitialCurrent=0  Capacitance=C  Setx0=on  InitialVoltage=V_voc_2  Measurements=None
  Product : Product
  Product1 : Product
  Square : Math  Operator=square
  Square1 : Math  Operator=square
  Subtract : Sum  Inputs=+-
  Voltage Measurement : spsVoltageMeasurementLib/Voltage Measurement  PhasorSimulation=off  OutputType=Complex  PSBequivalent=0
  val : Outport
  vbe : Outport  Port=2
  wires:
  Gain6/1 -> [im]
  Product1/1 -> Gain6/1
  [x1] -> Product1/2
  Gain5/1 -> [vm]
  Product/1 -> Gain5/1
  [x2] -> Product/2
  Subtract/1 -> Product/1, Product1/1
  Add/1 -> Subtract/2
  Square/1 -> Add/2
  Square1/1 -> Add/1
  Constant/1 -> Subtract/1
  Current Measurement/1 -> Gain4/1
  Gain4/1 -> Memory/1, Gain3/1
  Gain3/1 -> vbe/1
  [vm] -> Controlled Voltage Source1/1
  [im] -> Controlled Current Source1/1
  Gain2/1 -> Controlled Voltage Source2/1
  [u2] -> Gain2/1
  [u1] -> Controlled Current Source/1
  Demux/2 -> [u2]
  Demux/1 -> [u1]
  Gain/1 -> Demux/1
  Gain1/1 -> val/1
  Voltage Measurement/1 -> Memory1/1, Gain1/1
  u/1 -> Gain/1
  [x1] -> Square1/1
  [x2] -> Square/1
  Memory/1 -> [x2]
  Memory1/1 -> [x1]
  connections:
  Controlled Voltage Source2/LConn1 -- Current Measurement/LConn1
  Controlled Voltage Source2/RConn1 -- Controlled Voltage Source1/RConn1
  Controlled Voltage Source1/LConn1 -- Parallel RLC Branch1/RConn1
  Voltage Measurement/LConn1 -- Parallel RLC Branch2/LConn1 -- Parallel RLC Branch1/LConn1 -- Controlled Current Source1/RConn1 -- Controlled Current Source/LConn1
  Voltage Measurement/LConn2 -- Parallel RLC Branch2/RConn1 -- Current Measurement/RConn1 -- Controlled Current Source/RConn1 -- Controlled Current Source1/LConn1

== system PVAndBatteryIntegratedPlantForBlackStart_SPS/Battery Inverter/Inverter Control/VOC Control/Subsystem/rotate ==
  deltai : Inport
  Demux : Demux  Outputs=2
  Gain : Gain  Gain=-1
  Mux : Mux  Inputs=2
  u : Outport
  wires:
  deltai/1 -> Demux/1
  Mux/1 -> u/1
  Demux/2 -> Gain/1
  Gain/1 -> Mux/1
  Demux/1 -> Mux/2
